simulink model "Model_Simulation"  (R2018b)
settings: Solver=ode4  StartTime=0.0  StopTime=1600  FixedStep=1e-3  RelTol=1e-3
settings Model: Creator=auralius  LastModifiedBy=auralius

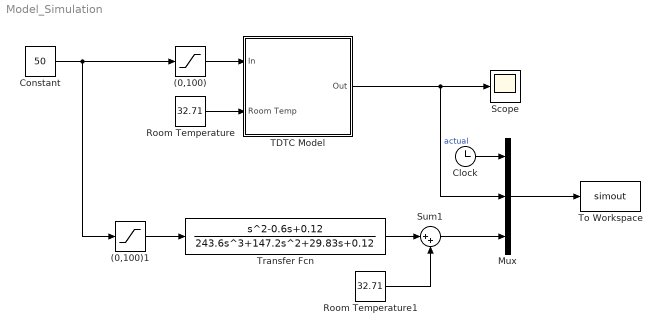
== system Model_Simulation ==
  (0,100) : Saturate  UpperLimit=100  LowerLimit=0
  (0,100)1 : Saturate  UpperLimit=100  LowerLimit=0
  Clock : Clock
  Constant : Constant  Value=50
  Mux : Mux  Inputs=3
  Room Temperature : Constant  Value=32.71
  Room Temperature1 : Constant  Value=32.71
  Scope : Scope
  Sum1 : Sum  Inputs=|++
  TDTC Model : Subsystem
  To Workspace : ToWorkspace  VariableName=simout  SampleTime=-1
  Transfer Fcn : TransferFcn  Numerator=[1 -0.6 0.12]  Denominator=[243.6 147.2 29.83 0.12]
  wires:
  Mux/1 -> To Workspace/1
  Clock/1 -> Mux/1
  TDTC Model/1(Out) -> Scope/1, Mux/2  "actual"
  (0,100)/1 -> TDTC Model/1(In)
  Room Temperature/1 -> TDTC Model/2(Room Temp)
  Room Temperature1/1 -> Sum1/2
  (0,100)1/1 -> Transfer Fcn/1
  Constant/1 -> (0,100)/1, (0,100)1/1
  Transfer Fcn/1 -> Sum1/1
  Sum1/1 -> Mux/3

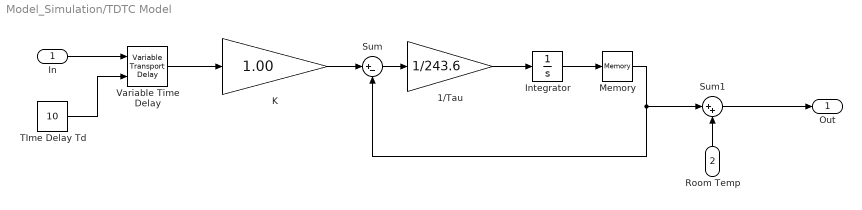
== system Model_Simulation/TDTC Model ==
  In : Inport
  Room Temp : Inport  Port=2
  1/Tau : Gain  Gain=1/243.6
  Integrator : Integrator
  K : Gain  Gain=1.00
  Memory : Memory
  Sum : Sum  Inputs=|+-
  Sum1 : Sum  Inputs=|++
  TIme Delay Td : Constant  Value=10
  Variable Time Delay : VariableTransportDelay  MaximumDelay=50
  Out : Outport
  wires:
  K/1 -> Sum/1
  Memory/1 -> Sum/2, Sum1/1
  In/1 -> Variable Time Delay/1
  Sum/1 -> 1/Tau/1
  Integrator/1 -> Memory/1
  Variable Time Delay/1 -> K/1
  Sum1/1 -> Out/1
  TIme Delay Td/1 -> Variable Time Delay/2
  1/Tau/1 -> Integrator/1
  Room Temp/1 -> Sum1/2
